simulink model "example_main_NDI_f16"  (R2020a)
settings: Solver=ode4  StartTime=0.0  StopTime=75  FixedStep=0.01  RelTol=1e-3
PreLoadFcn:
  | PreLoadFcn
values from neighbouring files (symbols this model uses):
  g = 32.17    [PreLoadFcn.m]
  N = [ 1      0     0.25 ... (first row only)    [PreLoadFcn.m]
  state0 = [IC.npos IC.epos IC.alt IC.q0 IC.q1 IC.q2 IC.q3  IC.p IC.q IC.r IC.alpha IC.beta IC.mu IC.Vt IC.chi IC.gamma]    [PreLoadFcn.m]
undefined symbols (not defined in the file or in its folder): Aactuator, ac, AeroCoeff, EngineTable, ft, IC, kg, m, Newton, PIController, Raphson, s, sigbuilder_block, slug
libraries: aerolibconvert2 x19, simulink x13, sharedutil x1
(part 1 of 6)
settings Model: Creator=User  LastModifiedBy=user
settings DataIOCC: ReturnWorkspaceOutputs=off
settings DebuggingCC: ArithmeticOperatorsInVariantConditions=warning
settings SFSimCC: CustomCodeUndefinedFunction=UseInterfaceOnly

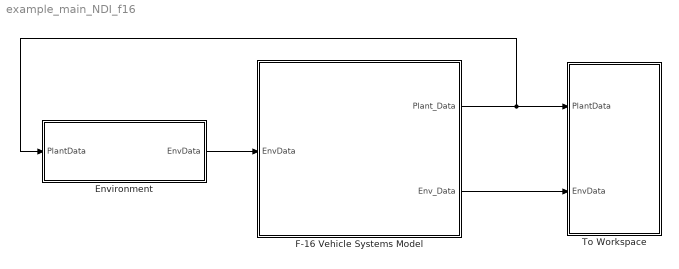
== system example_main_NDI_f16 ==
  Environment : Subsystem
      mask Display:
      | image('aeroenvironment.bmp','center')
      | % 左側 "Icon transparency" 欄位已選擇 "Opaque with ports"，所以埠名稱會自動顯示，不用再宣告
      | % port_label('input',1,'PlantData')
      | % port_label('output',1,'EnvData')
  F-16 Vehicle Systems Model : Subsystem
      mask Display:
      | image([pwd,'\image\wikipedia_F-16.jpg'],'center');
      | % 左側 "Icon transparency" 欄位已選擇 "Opaque with ports"，所以埠名稱會自動顯示，不用再宣告
      | % port_label('input',1,'EnvData')
      | % port_label('output',1,'Plant_Data')
      | % port_label('output',2,'Env_Data')
  To Workspace : Subsystem
  wires:
  F-16 Vehicle Systems Model/1(Plant_Data) -> To Workspace/1(PlantData), Environment/1(PlantData)
  Environment/1(EnvData) -> F-16 Vehicle Systems Model/1(EnvData)
  F-16 Vehicle Systems Model/2(Env_Data) -> To Workspace/2(EnvData)

== system example_main_NDI_f16/Environment ==
  PlantData : Inport
  "ISP " : Subsystem
  end5 : Terminator
  end8 : Terminator
  end9 : Terminator
  gravity (ft/s^2) : Constant  Value=g
  Out Bus Element : Outport  PortName=EnvData  Element=P
  Out Bus Element1 : Outport  PortName=EnvData  Element=AirDensity
  Out Bus Element2 : Outport  PortName=EnvData  Element=qbar
  Out Bus Element3 : Outport  PortName=EnvData  Element=Mach
  Out Bus Element4 : Outport  PortName=EnvData  Element=g
  wires:
  "ISP "/7(mu) -> end9/1
  "ISP "/5(T(K)) -> end5/1
  "ISP "/6(g (m/s^2)) -> end8/1
  PlantData/1 -> "ISP "/1(PlantData)
  "ISP "/1(P(HPa)) -> Out Bus Element/1
  "ISP "/2(rho(kg/m^3)) -> Out Bus Element1/1
  "ISP "/3(qbar (lbf/ft^2)) -> Out Bus Element2/1
  "ISP "/4("Mach ") -> Out Bus Element3/1
  gravity (ft/s^2)/1 -> Out Bus Element4/1  "g"

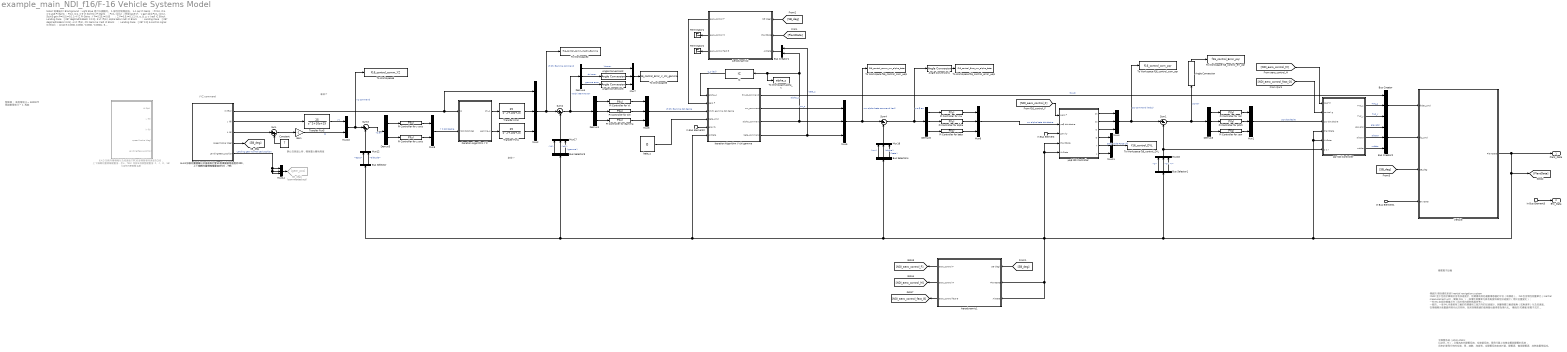
== system example_main_NDI_f16/F-16 Vehicle Systems Model ==
  note: 發動機：
      | 高度限制 0 ~ 50000 ft
      | 馬赫數限制 0 ~ 1 馬赫
  note: 全靜壓系統（pitot-static system），又稱為皮托靜壓系統、空速管系統，是飛行器上收集全壓與靜壓的系統，
      | 用來計算飛行時的空速、馬赫數、海拔等。全靜壓系統由皮托管、靜壓源、備用靜壓源、加熱裝置等組成。
  note: 傳統的 慣性導航系統(inertial navigation system (INS))至少包括計算機及含有加速度計、陀螺儀或其他運動傳感器的平台（或模組）。
      | INS包含慣性測量單元（Inertial measurement unit，簡稱 IMU ），該慣性測量單元具有角度和線性加速度計（用於位置變化）；
      | 一些IMU包括陀螺儀元件（用於保持絕對角度參考）。
      | 一般的，一個IMU內會裝有三軸的陀螺儀和三個方向的加速度計，測量物體三軸姿態角（或角速率）以及加速度。
      |
      | 在飛機顯示裝置變得現代化的同時，為其採集數據的感測器也變得更為現代化。
      | 傳統的 陀螺儀 被電子式的 航向姿態基準系統 （AHRS）與 大氣數據計算機 （ADC）所取代，
      | 在增加可靠性的同時也降低了成本、簡化了維護。
      | 此外， GPS 接收器也被整合進了玻璃駕駛艙之中。
  note: 機載電子設備
  note: 靜止在跑道上時，機身重心離地高度
  note: 拿掉!?
  note: VYZ command
  note: Note:(宥瑋論文)
      | Blockground：Light Blue 是可以調動的。
      | 1.線性控制增益值。
      | 1-1 pqr PI Gains：P=10, I=4.
      | 1-2 μαβ PI Gains：P=2, I=1.
      | 1-3 Vt $\chi$ γ PI Gains：P=1, I=0.2；降落Case:Vt、γ gain設定P=1, I=0.2、 $\chi$ gain P=0.5,I=0.1
      | 1-4 YZ PI Gains : Y P=0.25,I=0.05；Z P=0.5,I=0.1
      | 2.Vt, α, β, μ, γ (rad) IC Block
      | Landing Case：[287 deg2rad(9.8641) 0 0 0].
      | 3.Vt (ft/s), alpha beta (rad) IC Block：
      | Landing Case：[287 deg2rad(9.8641) 0.01].
      | 4.Vt (ft/s), Chi Gamma (rad) IC Block：
      | Landing Case：[287 0 0]
      | 5.control signal IC Block：
      | [2110 5 0.0001 0.0001 -0.0001 -0.0001].
      | 6. 若要在不同高度或是速度下飛行，需重新配平，以配平條件設定初始值。
      | 7. 控制分配權重值需在"pqr NDI Controller/innear NDI"中，N矩陣做調整。
      | 7. 減速板角度調整要在
      | "SB_Aerodynamic_coefficient"、"SB_Aerodynamic_coefficient_2017_iteration"、"SB_Aerodynamic_coefficient_2017_NDI"的m-file檔中做調整。
  note: 拿掉!?
  In Bus Element1 : Inport  PortName=EnvData
  In Bus Element3 : Inport  PortName=EnvData
  In Bus Element : Inport  PortName=EnvData  Element=g
  In Bus Element2 : Inport  PortName=EnvData  Element=g
  6.4.3加裝向量噴嘴以及減速版打開30度模擬著陸速度為200， 上下偏轉向量噴嘴權重值為4，75S (附錄B須調整權重值: 2、4、8、16) : Subsystem  Tag=STV Subsys  Commented=on  LoadFcn=sigbuilder_block('load');  StartFcn=sigbuilder_block('start');  StopFcn=sigbuilder_block('stop');  ClipboardFcn=sigbuilder_block('clipboard');  mask(Sigbuilder block){tuvar=[0:10]}
      mask help: Simulink:masks:SigbuilderBlock_MD
      mask init:
      | if ~strcmp(get_param(bdroot(gcbh),'SimulationStatus'),'stopped') tuvar = sigbuilder_block('maskInit'); end
      settings: CopyFcn=sigbuilder_block('copy');  DeleteFcn=sigbuilder_block('delete');  ModelCloseFcn=sigbuilder_block('modelClose');  PreSaveFcn=sigbuilder_block('preSave');  PauseFcn=sigbuilder_block('pause');  ContinueFcn=sigbuilder_block('continue');  NameChangeFcn=sigbuilder_block('namechange');  OpenFcn=sigbuilder_block('open',[6 30 1428 680.25 ]);  CloseFcn=sigbuilder_block('close');
      mask Display: plot(0, 0, 100, 100,[2, 2, 32, 32, 2], [68, 8, 8, 68, 68],[32, 2], [38, 38], [32, 19, 2],[53, 60, 44], [32, 17, 17, 2],[16, 16, 31, 31]);txt = getActiveGroup(gcbh);text(2, 100, txt,'verticalAlignment', 'top');
  6.4.3加裝向量噴嘴以及減速版打開40度模擬著陸速度為200， 上下偏轉向量噴嘴權重值為5.5，75S : Subsystem  Tag=STV Subsys  LoadFcn=sigbuilder_block('load');  StartFcn=sigbuilder_block('start');  StopFcn=sigbuilder_block('stop');  ClipboardFcn=sigbuilder_block('clipboard');  mask(Sigbuilder block){tuvar=[0:10]}
      mask help: Simulink:masks:SigbuilderBlock_MD
      mask init:
      | if ~strcmp(get_param(bdroot(gcbh),'SimulationStatus'),'stopped') tuvar = sigbuilder_block('maskInit'); end
      settings: CopyFcn=sigbuilder_block('copy');  DeleteFcn=sigbuilder_block('delete');  ModelCloseFcn=sigbuilder_block('modelClose');  PreSaveFcn=sigbuilder_block('preSave');  PauseFcn=sigbuilder_block('pause');  ContinueFcn=sigbuilder_block('continue');  NameChangeFcn=sigbuilder_block('namechange');  OpenFcn=sigbuilder_block('open',[6 30 1428 680.25 ]);  CloseFcn=sigbuilder_block('close');
      mask Display: plot(0, 0, 100, 100,[2, 2, 32, 32, 2], [68, 8, 8, 68, 68],[32, 2], [38, 38], [32, 19, 2],[53, 60, 44], [32, 17, 17, 2],[16, 16, 31, 31]);txt = getActiveGroup(gcbh);text(2, 100, txt,'verticalAlignment', 'top');
  Aerodynamic1 : Subsystem
  Aerodynamic2 : Subsystem
  Angle Conversion{,1..3} (4 alike) : aerolibconvert2/Angle Conversion  IU=rad  OU=deg
  Bus Creator : BusCreator  Inputs=3
  Bus Creator1 : BusCreator  Inputs=2
  Bus Creator2 : BusCreator  Inputs=3
  Bus Selector : BusSelector  OutputSignals=epos,altitude
  Bus Selector1 : BusSelector  OutputSignals=p,q,r
  Bus Selector3 : BusSelector  OutputSignals=Vt,chi,gamma
  Bus Selector4 : BusSelector  OutputSignals=mu,alpha,beta
  Constant : Constant  Value=7
  Demux{1,3..4,6} (4 alike) : Demux  Outputs=3
  Demux5 : Demux  Outputs=2
  Gain : Gain  Gain=-1
  IC : InitialCondition  Value=IC.alpha
  Iteration Algorithm V chi gamma : Subsystem
  Iteration Algorithm Y Z : Subsystem
  Mux{1..7,11,14,16..18} (12 alike) : Mux  Inputs=3
  Mux10 : Mux  Inputs=2
  Mux12 : Mux  Inputs=2
  Mux9 : Mux  Inputs=2
  PI Controller for Chi : simulink/Continuous/PID Controller  Controller=PI  Form=Parallel  TimeDomain=Continuous-time  UseExternalTs=off  SampleTime=-1  IntegratorMethod=Forward Euler  FilterMethod=Forward Euler  ControllerParametersSource=internal  P=PIController.chi.P  I=PIController.chi.I  D=0  UseFilter=on  N=100  TunerSelectOption=Transfer Function Based (PID Tuner App)  InitialConditionSource=internal  InitialConditionForIntegrator=0  InitialConditionForFilter=0  DifferentiatorICPrevScaledInput=0  ExternalReset=none  TrackingMode=off  Kt=1  LimitOutput=off  UpperSaturationLimit=inf  LowerSaturationLimit=-inf  LinearizeAsGain=on  AntiWindupMode=none  Kb=1  POutMin=[]  POutMax=[]  IOutMin=[]  IOutMax=[]  DOutMin=[]  DOutMax=[]  NOutMin=[]  NOutMax=[]  SumOutMin=[]  SumOutMax=[]  SaturationOutMin=[]  SaturationOutMax=[]  PParamMin=[]  PParamMax=[]  IParamMin=[]  IParamMax=[]  DParamMin=[]  DParamMax=[]  NParamMin=[]  NParamMax=[]  KbParamMin=[]  KbParamMax=[]  KtParamMin=[]  KtParamMax=[]  KbOutMin=[]  KbOutMax=[]  KtOutMin=[]  KtOutMax=[]  IntegratorOutMin=[]  IntegratorOutMax=[]  FilterOutMin=[]  FilterOutMax=[]  SumI1OutMin=[]  SumI1OutMax=[]  SumI2OutMin=[]  SumI2OutMax=[]  SumI3OutMin=[]  SumI3OutMax=[]  SumI4OutMin=[]  SumI4OutMax=[]  SumDOutMin=[]  SumDOutMax=[]  DifferentiatorOutMin=[]  DifferentiatorOutMax=[]  FilterDiffOutCoefMin=[]  FilterDiffOutCoefMax=[]  ReciprocalOutMin=[]  ReciprocalOutMax=[]  SumDenOutMin=[]  SumDenOutMax=[]  SumNumOutMin=[]  SumNumOutMax=[]  DivideOutMin=[]  DivideOutMax=[]  UdiffTsProdOutMin=[]  UdiffTsProdOutMax=[]  NTsProdOutMin=[]  NTsProdOutMax=[]  UintegralTsProdOutMin=[]  UintegralTsProdOutMax=[]  UngainTsProdOutMin=[]  UngainTsProdOutMax=[]  IntegratorContinuousStateAttributes=''  IntegratorStateMustResolveToSignalObject=off  IntegratorRTWStateStorageClass=Auto  FilterContinuousStateAttributes=''  FilterStateMustResolveToSignalObject=off  FilterRTWStateStorageClass=Auto  ParallelPVariant=InternalParameters  IdealPVariant=Disabled  IVariant=InternalParameters  DVariant=Disabled  IntegratorVariant=Continuous  SatVariant=Disabled  AWVariant=Passthrough  PCopyVariant=Disabled  TRVariant=Disabled  FdbkBlocksVariant=Forward  IdealPFdbkVariant=Disabled  SatFdbkVariant=Disabled  DerivativeFilterVariant=Disabled  NVariant=Disabled  NCopyVariant=Disabled_SignalSpec  FilterICVariant=Disabled  IntegratorICVariant=InternalICs  ExternalResetVariant=Disabled  TRSumVariant=Passthrough  SumFdbkVariant=Disabled  SumVariant=Sum_PI  TsampFilterVariant=InternalTs  TsampNgainVariant=Passthrough  TsampIntegralVariant=Passthrough
  PI Controller for Gamma : simulink/Continuous/PID Controller  Controller=PI  Form=Parallel  TimeDomain=Continuous-time  UseExternalTs=off  SampleTime=-1  IntegratorMethod=Forward Euler  FilterMethod=Forward Euler  ControllerParametersSource=internal  P=PIController.gamma.P  I=PIController.gamma.I  D=0  UseFilter=on  N=100  TunerSelectOption=Transfer Function Based (PID Tuner App)  InitialConditionSource=internal  InitialConditionForIntegrator=0  InitialConditionForFilter=0  DifferentiatorICPrevScaledInput=0  ExternalReset=none  TrackingMode=off  Kt=1  LimitOutput=off  UpperSaturationLimit=inf  LowerSaturationLimit=-inf  LinearizeAsGain=on  AntiWindupMode=none  Kb=1  POutMin=[]  POutMax=[]  IOutMin=[]  IOutMax=[]  DOutMin=[]  DOutMax=[]  NOutMin=[]  NOutMax=[]  SumOutMin=[]  SumOutMax=[]  SaturationOutMin=[]  SaturationOutMax=[]  PParamMin=[]  PParamMax=[]  IParamMin=[]  IParamMax=[]  DParamMin=[]  DParamMax=[]  NParamMin=[]  NParamMax=[]  KbParamMin=[]  KbParamMax=[]  KtParamMin=[]  KtParamMax=[]  KbOutMin=[]  KbOutMax=[]  KtOutMin=[]  KtOutMax=[]  IntegratorOutMin=[]  IntegratorOutMax=[]  FilterOutMin=[]  FilterOutMax=[]  SumI1OutMin=[]  SumI1OutMax=[]  SumI2OutMin=[]  SumI2OutMax=[]  SumI3OutMin=[]  SumI3OutMax=[]  SumI4OutMin=[]  SumI4OutMax=[]  SumDOutMin=[]  SumDOutMax=[]  DifferentiatorOutMin=[]  DifferentiatorOutMax=[]  FilterDiffOutCoefMin=[]  FilterDiffOutCoefMax=[]  ReciprocalOutMin=[]  ReciprocalOutMax=[]  SumDenOutMin=[]  SumDenOutMax=[]  SumNumOutMin=[]  SumNumOutMax=[]  DivideOutMin=[]  DivideOutMax=[]  UdiffTsProdOutMin=[]  UdiffTsProdOutMax=[]  NTsProdOutMin=[]  NTsProdOutMax=[]  UintegralTsProdOutMin=[]  UintegralTsProdOutMax=[]  UngainTsProdOutMin=[]  UngainTsProdOutMax=[]  IntegratorContinuousStateAttributes=''  IntegratorStateMustResolveToSignalObject=off  IntegratorRTWStateStorageClass=Auto  FilterContinuousStateAttributes=''  FilterStateMustResolveToSignalObject=off  FilterRTWStateStorageClass=Auto  ParallelPVariant=InternalParameters  IdealPVariant=Disabled  IVariant=InternalParameters  DVariant=Disabled  IntegratorVariant=Continuous  SatVariant=Disabled  AWVariant=Passthrough  PCopyVariant=Disabled  TRVariant=Disabled  FdbkBlocksVariant=Forward  IdealPFdbkVariant=Disabled  SatFdbkVariant=Disabled  DerivativeFilterVariant=Disabled  NVariant=Disabled  NCopyVariant=Disabled_SignalSpec  FilterICVariant=Disabled  IntegratorICVariant=InternalICs  ExternalResetVariant=Disabled  TRSumVariant=Passthrough  SumFdbkVariant=Disabled  SumVariant=Sum_PI  TsampFilterVariant=InternalTs  TsampNgainVariant=Passthrough  TsampIntegralVariant=Passthrough
  PI Controller for Vt : simulink/Continuous/PID Controller  Controller=PI  Form=Parallel  TimeDomain=Continuous-time  UseExternalTs=off  SampleTime=-1  IntegratorMethod=Forward Euler  FilterMethod=Forward Euler  ControllerParametersSource=internal  P=PIController.Vt.P  I=PIController.Vt.I  D=0  UseFilter=on  N=100  TunerSelectOption=Transfer Function Based (PID Tuner App)  InitialConditionSource=internal  InitialConditionForIntegrator=0  InitialConditionForFilter=0  DifferentiatorICPrevScaledInput=0  ExternalReset=none  TrackingMode=off  Kt=1  LimitOutput=off  UpperSaturationLimit=inf  LowerSaturationLimit=-inf  LinearizeAsGain=on  AntiWindupMode=none  Kb=1  POutMin=[]  POutMax=[]  IOutMin=[]  IOutMax=[]  DOutMin=[]  DOutMax=[]  NOutMin=[]  NOutMax=[]  SumOutMin=[]  SumOutMax=[]  SaturationOutMin=[]  SaturationOutMax=[]  PParamMin=[]  PParamMax=[]  IParamMin=[]  IParamMax=[]  DParamMin=[]  DParamMax=[]  NParamMin=[]  NParamMax=[]  KbParamMin=[]  KbParamMax=[]  KtParamMin=[]  KtParamMax=[]  KbOutMin=[]  KbOutMax=[]  KtOutMin=[]  KtOutMax=[]  IntegratorOutMin=[]  IntegratorOutMax=[]  FilterOutMin=[]  FilterOutMax=[]  SumI1OutMin=[]  SumI1OutMax=[]  SumI2OutMin=[]  SumI2OutMax=[]  SumI3OutMin=[]  SumI3OutMax=[]  SumI4OutMin=[]  SumI4OutMax=[]  SumDOutMin=[]  SumDOutMax=[]  DifferentiatorOutMin=[]  DifferentiatorOutMax=[]  FilterDiffOutCoefMin=[]  FilterDiffOutCoefMax=[]  ReciprocalOutMin=[]  ReciprocalOutMax=[]  SumDenOutMin=[]  SumDenOutMax=[]  SumNumOutMin=[]  SumNumOutMax=[]  DivideOutMin=[]  DivideOutMax=[]  UdiffTsProdOutMin=[]  UdiffTsProdOutMax=[]  NTsProdOutMin=[]  NTsProdOutMax=[]  UintegralTsProdOutMin=[]  UintegralTsProdOutMax=[]  UngainTsProdOutMin=[]  UngainTsProdOutMax=[]  IntegratorContinuousStateAttributes=''  IntegratorStateMustResolveToSignalObject=off  IntegratorRTWStateStorageClass=Auto  FilterContinuousStateAttributes=''  FilterStateMustResolveToSignalObject=off  FilterRTWStateStorageClass=Auto  ParallelPVariant=InternalParameters  IdealPVariant=Disabled  IVariant=InternalParameters  DVariant=Disabled  IntegratorVariant=Continuous  SatVariant=Disabled  AWVariant=Passthrough  PCopyVariant=Disabled  TRVariant=Disabled  FdbkBlocksVariant=Forward  IdealPFdbkVariant=Disabled  SatFdbkVariant=Disabled  DerivativeFilterVariant=Disabled  NVariant=Disabled  NCopyVariant=Disabled_SignalSpec  FilterICVariant=Disabled  IntegratorICVariant=InternalICs  ExternalResetVariant=Disabled  TRSumVariant=Passthrough  SumFdbkVariant=Disabled  SumVariant=Sum_PI  TsampFilterVariant=InternalTs  TsampNgainVariant=Passthrough  TsampIntegralVariant=Passthrough
  PI Controller for alpha : simulink/Continuous/PID Controller  Controller=PI  Form=Parallel  TimeDomain=Continuous-time  UseExternalTs=off  SampleTime=-1  IntegratorMethod=Forward Euler  FilterMethod=Forward Euler  ControllerParametersSource=internal  P=PIController.alpha.P  I=PIController.alpha.I  D=0  UseFilter=on  N=100  TunerSelectOption=Transfer Function Based (PID Tuner App)  InitialConditionSource=internal  InitialConditionForIntegrator=0  InitialConditionForFilter=0  DifferentiatorICPrevScaledInput=0  ExternalReset=none  TrackingMode=off  Kt=1  LimitOutput=off  UpperSaturationLimit=inf  LowerSaturationLimit=-inf  LinearizeAsGain=on  AntiWindupMode=none  Kb=1  POutMin=[]  POutMax=[]  IOutMin=[]  IOutMax=[]  DOutMin=[]  DOutMax=[]  NOutMin=[]  NOutMax=[]  SumOutMin=[]  SumOutMax=[]  SaturationOutMin=[]  SaturationOutMax=[]  PParamMin=[]  PParamMax=[]  IParamMin=[]  IParamMax=[]  DParamMin=[]  DParamMax=[]  NParamMin=[]  NParamMax=[]  KbParamMin=[]  KbParamMax=[]  KtParamMin=[]  KtParamMax=[]  KbOutMin=[]  KbOutMax=[]  KtOutMin=[]  KtOutMax=[]  IntegratorOutMin=[]  IntegratorOutMax=[]  FilterOutMin=[]  FilterOutMax=[]  SumI1OutMin=[]  SumI1OutMax=[]  SumI2OutMin=[]  SumI2OutMax=[]  SumI3OutMin=[]  SumI3OutMax=[]  SumI4OutMin=[]  SumI4OutMax=[]  SumDOutMin=[]  SumDOutMax=[]  DifferentiatorOutMin=[]  DifferentiatorOutMax=[]  FilterDiffOutCoefMin=[]  FilterDiffOutCoefMax=[]  ReciprocalOutMin=[]  ReciprocalOutMax=[]  SumDenOutMin=[]  SumDenOutMax=[]  SumNumOutMin=[]  SumNumOutMax=[]  DivideOutMin=[]  DivideOutMax=[]  UdiffTsProdOutMin=[]  UdiffTsProdOutMax=[]  NTsProdOutMin=[]  NTsProdOutMax=[]  UintegralTsProdOutMin=[]  UintegralTsProdOutMax=[]  UngainTsProdOutMin=[]  UngainTsProdOutMax=[]  IntegratorContinuousStateAttributes=''  IntegratorStateMustResolveToSignalObject=off  IntegratorRTWStateStorageClass=Auto  FilterContinuousStateAttributes=''  FilterStateMustResolveToSignalObject=off  FilterRTWStateStorageClass=Auto  ParallelPVariant=InternalParameters  IdealPVariant=Disabled  IVariant=InternalParameters  DVariant=Disabled  IntegratorVariant=Continuous  SatVariant=Disabled  AWVariant=Passthrough  PCopyVariant=Disabled  TRVariant=Disabled  FdbkBlocksVariant=Forward  IdealPFdbkVariant=Disabled  SatFdbkVariant=Disabled  DerivativeFilterVariant=Disabled  NVariant=Disabled  NCopyVariant=Disabled_SignalSpec  FilterICVariant=Disabled  IntegratorICVariant=InternalICs  ExternalResetVariant=Disabled  TRSumVariant=Passthrough  SumFdbkVariant=Disabled  SumVariant=Sum_PI  TsampFilterVariant=InternalTs  TsampNgainVariant=Passthrough  TsampIntegralVariant=Passthrough
  PI Controller for beta : simulink/Continuous/PID Controller  Controller=PI  Form=Parallel  TimeDomain=Continuous-time  UseExternalTs=off  SampleTime=-1  IntegratorMethod=Forward Euler  FilterMethod=Forward Euler  ControllerParametersSource=internal  P=PIController.beta.P  I=PIController.beta.I  D=0  UseFilter=on  N=100  TunerSelectOption=Transfer Function Based (PID Tuner App)  InitialConditionSource=internal  InitialConditionForIntegrator=0  InitialConditionForFilter=0  DifferentiatorICPrevScaledInput=0  ExternalReset=none  TrackingMode=off  Kt=1  LimitOutput=off  UpperSaturationLimit=inf  LowerSaturationLimit=-inf  LinearizeAsGain=on  AntiWindupMode=none  Kb=1  POutMin=[]  POutMax=[]  IOutMin=[]  IOutMax=[]  DOutMin=[]  DOutMax=[]  NOutMin=[]  NOutMax=[]  SumOutMin=[]  SumOutMax=[]  SaturationOutMin=[]  SaturationOutMax=[]  PParamMin=[]  PParamMax=[]  IParamMin=[]  IParamMax=[]  DParamMin=[]  DParamMax=[]  NParamMin=[]  NParamMax=[]  KbParamMin=[]  KbParamMax=[]  KtParamMin=[]  KtParamMax=[]  KbOutMin=[]  KbOutMax=[]  KtOutMin=[]  KtOutMax=[]  IntegratorOutMin=[]  IntegratorOutMax=[]  FilterOutMin=[]  FilterOutMax=[]  SumI1OutMin=[]  SumI1OutMax=[]  SumI2OutMin=[]  SumI2OutMax=[]  SumI3OutMin=[]  SumI3OutMax=[]  SumI4OutMin=[]  SumI4OutMax=[]  SumDOutMin=[]  SumDOutMax=[]  DifferentiatorOutMin=[]  DifferentiatorOutMax=[]  FilterDiffOutCoefMin=[]  FilterDiffOutCoefMax=[]  ReciprocalOutMin=[]  ReciprocalOutMax=[]  SumDenOutMin=[]  SumDenOutMax=[]  SumNumOutMin=[]  SumNumOutMax=[]  DivideOutMin=[]  DivideOutMax=[]  UdiffTsProdOutMin=[]  UdiffTsProdOutMax=[]  NTsProdOutMin=[]  NTsProdOutMax=[]  UintegralTsProdOutMin=[]  UintegralTsProdOutMax=[]  UngainTsProdOutMin=[]  UngainTsProdOutMax=[]  IntegratorContinuousStateAttributes=''  IntegratorStateMustResolveToSignalObject=off  IntegratorRTWStateStorageClass=Auto  FilterContinuousStateAttributes=''  FilterStateMustResolveToSignalObject=off  FilterRTWStateStorageClass=Auto  ParallelPVariant=InternalParameters  IdealPVariant=Disabled  IVariant=InternalParameters  DVariant=Disabled  IntegratorVariant=Continuous  SatVariant=Disabled  AWVariant=Passthrough  PCopyVariant=Disabled  TRVariant=Disabled  FdbkBlocksVariant=Forward  IdealPFdbkVariant=Disabled  SatFdbkVariant=Disabled  DerivativeFilterVariant=Disabled  NVariant=Disabled  NCopyVariant=Disabled_SignalSpec  FilterICVariant=Disabled  IntegratorICVariant=InternalICs  ExternalResetVariant=Disabled  TRSumVariant=Passthrough  SumFdbkVariant=Disabled  SumVariant=Sum_PI  TsampFilterVariant=InternalTs  TsampNgainVariant=Passthrough  TsampIntegralVariant=Passthrough
  PI Controller for mu : simulink/Continuous/PID Controller  Controller=PI  Form=Parallel  TimeDomain=Continuous-time  UseExternalTs=off  SampleTime=-1  IntegratorMethod=Forward Euler  FilterMethod=Forward Euler  ControllerParametersSource=internal  P=PIController.mu.P  I=PIController.mu.I  D=0  UseFilter=on  N=100  TunerSelectOption=Transfer Function Based (PID Tuner App)  InitialConditionSource=internal  InitialConditionForIntegrator=0  InitialConditionForFilter=0  DifferentiatorICPrevScaledInput=0  ExternalReset=none  TrackingMode=off  Kt=1  LimitOutput=off  UpperSaturationLimit=inf  LowerSaturationLimit=-inf  LinearizeAsGain=on  AntiWindupMode=none  Kb=1  POutMin=[]  POutMax=[]  IOutMin=[]  IOutMax=[]  DOutMin=[]  DOutMax=[]  NOutMin=[]  NOutMax=[]  SumOutMin=[]  SumOutMax=[]  SaturationOutMin=[]  SaturationOutMax=[]  PParamMin=[]  PParamMax=[]  IParamMin=[]  IParamMax=[]  DParamMin=[]  DParamMax=[]  NParamMin=[]  NParamMax=[]  KbParamMin=[]  KbParamMax=[]  KtParamMin=[]  KtParamMax=[]  KbOutMin=[]  KbOutMax=[]  KtOutMin=[]  KtOutMax=[]  IntegratorOutMin=[]  IntegratorOutMax=[]  FilterOutMin=[]  FilterOutMax=[]  SumI1OutMin=[]  SumI1OutMax=[]  SumI2OutMin=[]  SumI2OutMax=[]  SumI3OutMin=[]  SumI3OutMax=[]  SumI4OutMin=[]  SumI4OutMax=[]  SumDOutMin=[]  SumDOutMax=[]  DifferentiatorOutMin=[]  DifferentiatorOutMax=[]  FilterDiffOutCoefMin=[]  FilterDiffOutCoefMax=[]  ReciprocalOutMin=[]  ReciprocalOutMax=[]  SumDenOutMin=[]  SumDenOutMax=[]  SumNumOutMin=[]  SumNumOutMax=[]  DivideOutMin=[]  DivideOutMax=[]  UdiffTsProdOutMin=[]  UdiffTsProdOutMax=[]  NTsProdOutMin=[]  NTsProdOutMax=[]  UintegralTsProdOutMin=[]  UintegralTsProdOutMax=[]  UngainTsProdOutMin=[]  UngainTsProdOutMax=[]  IntegratorContinuousStateAttributes=''  IntegratorStateMustResolveToSignalObject=off  IntegratorRTWStateStorageClass=Auto  FilterContinuousStateAttributes=''  FilterStateMustResolveToSignalObject=off  FilterRTWStateStorageClass=Auto  ParallelPVariant=InternalParameters  IdealPVariant=Disabled  IVariant=InternalParameters  DVariant=Disabled  IntegratorVariant=Continuous  SatVariant=Disabled  AWVariant=Passthrough  PCopyVariant=Disabled  TRVariant=Disabled  FdbkBlocksVariant=Forward  IdealPFdbkVariant=Disabled  SatFdbkVariant=Disabled  DerivativeFilterVariant=Disabled  NVariant=Disabled  NCopyVariant=Disabled_SignalSpec  FilterICVariant=Disabled  IntegratorICVariant=InternalICs  ExternalResetVariant=Disabled  TRSumVariant=Passthrough  SumFdbkVariant=Disabled  SumVariant=Sum_PI  TsampFilterVariant=InternalTs  TsampNgainVariant=Passthrough  TsampIntegralVariant=Passthrough
  PI Controller for pitch : simulink/Continuous/PID Controller  Controller=PI  Form=Parallel  TimeDomain=Continuous-time  UseExternalTs=off  SampleTime=-1  IntegratorMethod=Forward Euler  FilterMethod=Forward Euler  ControllerParametersSource=internal  P=PIController.q.P  I=PIController.q.I  D=0  UseFilter=on  N=100  TunerSelectOption=Transfer Function Based (PID Tuner App)  InitialConditionSource=internal  InitialConditionForIntegrator=0  InitialConditionForFilter=0  DifferentiatorICPrevScaledInput=0  ExternalReset=none  TrackingMode=off  Kt=1  LimitOutput=off  UpperSaturationLimit=inf  LowerSaturationLimit=-inf  LinearizeAsGain=on  AntiWindupMode=none  Kb=1  POutMin=[]  POutMax=[]  IOutMin=[]  IOutMax=[]  DOutMin=[]  DOutMax=[]  NOutMin=[]  NOutMax=[]  SumOutMin=[]  SumOutMax=[]  SaturationOutMin=[]  SaturationOutMax=[]  PParamMin=[]  PParamMax=[]  IParamMin=[]  IParamMax=[]  DParamMin=[]  DParamMax=[]  NParamMin=[]  NParamMax=[]  KbParamMin=[]  KbParamMax=[]  KtParamMin=[]  KtParamMax=[]  KbOutMin=[]  KbOutMax=[]  KtOutMin=[]  KtOutMax=[]  IntegratorOutMin=[]  IntegratorOutMax=[]  FilterOutMin=[]  FilterOutMax=[]  SumI1OutMin=[]  SumI1OutMax=[]  SumI2OutMin=[]  SumI2OutMax=[]  SumI3OutMin=[]  SumI3OutMax=[]  SumI4OutMin=[]  SumI4OutMax=[]  SumDOutMin=[]  SumDOutMax=[]  DifferentiatorOutMin=[]  DifferentiatorOutMax=[]  FilterDiffOutCoefMin=[]  FilterDiffOutCoefMax=[]  ReciprocalOutMin=[]  ReciprocalOutMax=[]  SumDenOutMin=[]  SumDenOutMax=[]  SumNumOutMin=[]  SumNumOutMax=[]  DivideOutMin=[]  DivideOutMax=[]  UdiffTsProdOutMin=[]  UdiffTsProdOutMax=[]  NTsProdOutMin=[]  NTsProdOutMax=[]  UintegralTsProdOutMin=[]  UintegralTsProdOutMax=[]  UngainTsProdOutMin=[]  UngainTsProdOutMax=[]  IntegratorContinuousStateAttributes=''  IntegratorStateMustResolveToSignalObject=off  IntegratorRTWStateStorageClass=Auto  FilterContinuousStateAttributes=''  FilterStateMustResolveToSignalObject=off  FilterRTWStateStorageClass=Auto  ParallelPVariant=InternalParameters  IdealPVariant=Disabled  IVariant=InternalParameters  DVariant=Disabled  IntegratorVariant=Continuous  SatVariant=Disabled  AWVariant=Passthrough  PCopyVariant=Disabled  TRVariant=Disabled  FdbkBlocksVariant=Forward  IdealPFdbkVariant=Disabled  SatFdbkVariant=Disabled  DerivativeFilterVariant=Disabled  NVariant=Disabled  NCopyVariant=Disabled_SignalSpec  FilterICVariant=Disabled  IntegratorICVariant=InternalICs  ExternalResetVariant=Disabled  TRSumVariant=Passthrough  SumFdbkVariant=Disabled  SumVariant=Sum_PI  TsampFilterVariant=InternalTs  TsampNgainVariant=Passthrough  TsampIntegralVariant=Passthrough
  PI Controller for roll : simulink/Continuous/PID Controller  Controller=PI  Form=Parallel  TimeDomain=Continuous-time  UseExternalTs=off  SampleTime=-1  IntegratorMethod=Forward Euler  FilterMethod=Forward Euler  ControllerParametersSource=internal  P=PIController.p.P  I=PIController.p.I  D=0  UseFilter=on  N=100  TunerSelectOption=Transfer Function Based (PID Tuner App)  InitialConditionSource=internal  InitialConditionForIntegrator=0  InitialConditionForFilter=0  DifferentiatorICPrevScaledInput=0  ExternalReset=none  TrackingMode=off  Kt=1  LimitOutput=off  UpperSaturationLimit=inf  LowerSaturationLimit=-inf  LinearizeAsGain=on  AntiWindupMode=none  Kb=1  POutMin=[]  POutMax=[]  IOutMin=[]  IOutMax=[]  DOutMin=[]  DOutMax=[]  NOutMin=[]  NOutMax=[]  SumOutMin=[]  SumOutMax=[]  SaturationOutMin=[]  SaturationOutMax=[]  PParamMin=[]  PParamMax=[]  IParamMin=[]  IParamMax=[]  DParamMin=[]  DParamMax=[]  NParamMin=[]  NParamMax=[]  KbParamMin=[]  KbParamMax=[]  KtParamMin=[]  KtParamMax=[]  KbOutMin=[]  KbOutMax=[]  KtOutMin=[]  KtOutMax=[]  IntegratorOutMin=[]  IntegratorOutMax=[]  FilterOutMin=[]  FilterOutMax=[]  SumI1OutMin=[]  SumI1OutMax=[]  SumI2OutMin=[]  SumI2OutMax=[]  SumI3OutMin=[]  SumI3OutMax=[]  SumI4OutMin=[]  SumI4OutMax=[]  SumDOutMin=[]  SumDOutMax=[]  DifferentiatorOutMin=[]  DifferentiatorOutMax=[]  FilterDiffOutCoefMin=[]  FilterDiffOutCoefMax=[]  ReciprocalOutMin=[]  ReciprocalOutMax=[]  SumDenOutMin=[]  SumDenOutMax=[]  SumNumOutMin=[]  SumNumOutMax=[]  DivideOutMin=[]  DivideOutMax=[]  UdiffTsProdOutMin=[]  UdiffTsProdOutMax=[]  NTsProdOutMin=[]  NTsProdOutMax=[]  UintegralTsProdOutMin=[]  UintegralTsProdOutMax=[]  UngainTsProdOutMin=[]  UngainTsProdOutMax=[]  IntegratorContinuousStateAttributes=''  IntegratorStateMustResolveToSignalObject=off  IntegratorRTWStateStorageClass=Auto  FilterContinuousStateAttributes=''  FilterStateMustResolveToSignalObject=off  FilterRTWStateStorageClass=Auto  ParallelPVariant=InternalParameters  IdealPVariant=Disabled  IVariant=InternalParameters  DVariant=Disabled  IntegratorVariant=Continuous  SatVariant=Disabled  AWVariant=Passthrough  PCopyVariant=Disabled  TRVariant=Disabled  FdbkBlocksVariant=Forward  IdealPFdbkVariant=Disabled  SatFdbkVariant=Disabled  DerivativeFilterVariant=Disabled  NVariant=Disabled  NCopyVariant=Disabled_SignalSpec  FilterICVariant=Disabled  IntegratorICVariant=InternalICs  ExternalResetVariant=Disabled  TRSumVariant=Passthrough  SumFdbkVariant=Disabled  SumVariant=Sum_PI  TsampFilterVariant=InternalTs  TsampNgainVariant=Passthrough  TsampIntegralVariant=Passthrough
  PI Controller for y axis : simulink/Continuous/PID Controller  Controller=PI  Form=Parallel  TimeDomain=Continuous-time  UseExternalTs=off  SampleTime=-1  IntegratorMethod=Forward Euler  FilterMethod=Forward Euler  ControllerParametersSource=internal  P=PIController.y.P  I=PIController.y.I  D=0  UseFilter=on  N=100  TunerSelectOption=Transfer Function Based (PID Tuner App)  InitialConditionSource=internal  InitialConditionForIntegrator=0  InitialConditionForFilter=0  DifferentiatorICPrevScaledInput=0  ExternalReset=none  TrackingMode=off  Kt=1  LimitOutput=off  UpperSaturationLimit=inf  LowerSaturationLimit=-inf  LinearizeAsGain=on  AntiWindupMode=none  Kb=1  POutMin=[]  POutMax=[]  IOutMin=[]  IOutMax=[]  DOutMin=[]  DOutMax=[]  NOutMin=[]  NOutMax=[]  SumOutMin=[]  SumOutMax=[]  SaturationOutMin=[]  SaturationOutMax=[]  PParamMin=[]  PParamMax=[]  IParamMin=[]  IParamMax=[]  DParamMin=[]  DParamMax=[]  NParamMin=[]  NParamMax=[]  KbParamMin=[]  KbParamMax=[]  KtParamMin=[]  KtParamMax=[]  KbOutMin=[]  KbOutMax=[]  KtOutMin=[]  KtOutMax=[]  IntegratorOutMin=[]  IntegratorOutMax=[]  FilterOutMin=[]  FilterOutMax=[]  SumI1OutMin=[]  SumI1OutMax=[]  SumI2OutMin=[]  SumI2OutMax=[]  SumI3OutMin=[]  SumI3OutMax=[]  SumI4OutMin=[]  SumI4OutMax=[]  SumDOutMin=[]  SumDOutMax=[]  DifferentiatorOutMin=[]  DifferentiatorOutMax=[]  FilterDiffOutCoefMin=[]  FilterDiffOutCoefMax=[]  ReciprocalOutMin=[]  ReciprocalOutMax=[]  SumDenOutMin=[]  SumDenOutMax=[]  SumNumOutMin=[]  SumNumOutMax=[]  DivideOutMin=[]  DivideOutMax=[]  UdiffTsProdOutMin=[]  UdiffTsProdOutMax=[]  NTsProdOutMin=[]  NTsProdOutMax=[]  UintegralTsProdOutMin=[]  UintegralTsProdOutMax=[]  UngainTsProdOutMin=[]  UngainTsProdOutMax=[]  IntegratorContinuousStateAttributes=''  IntegratorStateMustResolveToSignalObject=off  IntegratorRTWStateStorageClass=Auto  FilterContinuousStateAttributes=''  FilterStateMustResolveToSignalObject=off  FilterRTWStateStorageClass=Auto  ParallelPVariant=InternalParameters  IdealPVariant=Disabled  IVariant=InternalParameters  DVariant=Disabled  IntegratorVariant=Continuous  SatVariant=Disabled  AWVariant=Passthrough  PCopyVariant=Disabled  TRVariant=Disabled  FdbkBlocksVariant=Forward  IdealPFdbkVariant=Disabled  SatFdbkVariant=Disabled  DerivativeFilterVariant=Disabled  NVariant=Disabled  NCopyVariant=Disabled_SignalSpec  FilterICVariant=Disabled  IntegratorICVariant=InternalICs  ExternalResetVariant=Disabled  TRSumVariant=Passthrough  SumFdbkVariant=Disabled  SumVariant=Sum_PI  TsampFilterVariant=InternalTs  TsampNgainVariant=Passthrough  TsampIntegralVariant=Passthrough
  PI Controller for yaw : simulink/Continuous/PID Controller  Controller=PI  Form=Parallel  TimeDomain=Continuous-time  UseExternalTs=off  SampleTime=-1  IntegratorMethod=Forward Euler  FilterMethod=Forward Euler  ControllerParametersSource=internal  P=PIController.r.P  I=PIController.r.I  D=0  UseFilter=on  N=100  TunerSelectOption=Transfer Function Based (PID Tuner App)  InitialConditionSource=internal  InitialConditionForIntegrator=0  InitialConditionForFilter=0  DifferentiatorICPrevScaledInput=0  ExternalReset=none  TrackingMode=off  Kt=1  LimitOutput=off  UpperSaturationLimit=inf  LowerSaturationLimit=-inf  LinearizeAsGain=on  AntiWindupMode=none  Kb=1  POutMin=[]  POutMax=[]  IOutMin=[]  IOutMax=[]  DOutMin=[]  DOutMax=[]  NOutMin=[]  NOutMax=[]  SumOutMin=[]  SumOutMax=[]  SaturationOutMin=[]  SaturationOutMax=[]  PParamMin=[]  PParamMax=[]  IParamMin=[]  IParamMax=[]  DParamMin=[]  DParamMax=[]  NParamMin=[]  NParamMax=[]  KbParamMin=[]  KbParamMax=[]  KtParamMin=[]  KtParamMax=[]  KbOutMin=[]  KbOutMax=[]  KtOutMin=[]  KtOutMax=[]  IntegratorOutMin=[]  IntegratorOutMax=[]  FilterOutMin=[]  FilterOutMax=[]  SumI1OutMin=[]  SumI1OutMax=[]  SumI2OutMin=[]  SumI2OutMax=[]  SumI3OutMin=[]  SumI3OutMax=[]  SumI4OutMin=[]  SumI4OutMax=[]  SumDOutMin=[]  SumDOutMax=[]  DifferentiatorOutMin=[]  DifferentiatorOutMax=[]  FilterDiffOutCoefMin=[]  FilterDiffOutCoefMax=[]  ReciprocalOutMin=[]  ReciprocalOutMax=[]  SumDenOutMin=[]  SumDenOutMax=[]  SumNumOutMin=[]  SumNumOutMax=[]  DivideOutMin=[]  DivideOutMax=[]  UdiffTsProdOutMin=[]  UdiffTsProdOutMax=[]  NTsProdOutMin=[]  NTsProdOutMax=[]  UintegralTsProdOutMin=[]  UintegralTsProdOutMax=[]  UngainTsProdOutMin=[]  UngainTsProdOutMax=[]  IntegratorContinuousStateAttributes=''  IntegratorStateMustResolveToSignalObject=off  IntegratorRTWStateStorageClass=Auto  FilterContinuousStateAttributes=''  FilterStateMustResolveToSignalObject=off  FilterRTWStateStorageClass=Auto  ParallelPVariant=InternalParameters  IdealPVariant=Disabled  IVariant=InternalParameters  DVariant=Disabled  IntegratorVariant=Continuous  SatVariant=Disabled  AWVariant=Passthrough  PCopyVariant=Disabled  TRVariant=Disabled  FdbkBlocksVariant=Forward  IdealPFdbkVariant=Disabled  SatFdbkVariant=Disabled  DerivativeFilterVariant=Disabled  NVariant=Disabled  NCopyVariant=Disabled_SignalSpec  FilterICVariant=Disabled  IntegratorICVariant=InternalICs  ExternalResetVariant=Disabled  TRSumVariant=Passthrough  SumFdbkVariant=Disabled  SumVariant=Sum_PI  TsampFilterVariant=InternalTs  TsampNgainVariant=Passthrough  TsampIntegralVariant=Passthrough
  PI Controller for z axis : simulink/Continuous/PID Controller  Controller=PI  Form=Parallel  TimeDomain=Continuous-time  UseExternalTs=off  SampleTime=-1  IntegratorMethod=Forward Euler  FilterMethod=Forward Euler  ControllerParametersSource=internal  P=PIController.z.P  I=PIController.z.I  D=0  UseFilter=on  N=100  TunerSelectOption=Transfer Function Based (PID Tuner App)  InitialConditionSource=internal  InitialConditionForIntegrator=0  InitialConditionForFilter=0  DifferentiatorICPrevScaledInput=0  ExternalReset=none  TrackingMode=off  Kt=1  LimitOutput=off  UpperSaturationLimit=inf  LowerSaturationLimit=-inf  LinearizeAsGain=on  AntiWindupMode=none  Kb=1  POutMin=[]  POutMax=[]  IOutMin=[]  IOutMax=[]  DOutMin=[]  DOutMax=[]  NOutMin=[]  NOutMax=[]  SumOutMin=[]  SumOutMax=[]  SaturationOutMin=[]  SaturationOutMax=[]  PParamMin=[]  PParamMax=[]  IParamMin=[]  IParamMax=[]  DParamMin=[]  DParamMax=[]  NParamMin=[]  NParamMax=[]  KbParamMin=[]  KbParamMax=[]  KtParamMin=[]  KtParamMax=[]  KbOutMin=[]  KbOutMax=[]  KtOutMin=[]  KtOutMax=[]  IntegratorOutMin=[]  IntegratorOutMax=[]  FilterOutMin=[]  FilterOutMax=[]  SumI1OutMin=[]  SumI1OutMax=[]  SumI2OutMin=[]  SumI2OutMax=[]  SumI3OutMin=[]  SumI3OutMax=[]  SumI4OutMin=[]  SumI4OutMax=[]  SumDOutMin=[]  SumDOutMax=[]  DifferentiatorOutMin=[]  DifferentiatorOutMax=[]  FilterDiffOutCoefMin=[]  FilterDiffOutCoefMax=[]  ReciprocalOutMin=[]  ReciprocalOutMax=[]  SumDenOutMin=[]  SumDenOutMax=[]  SumNumOutMin=[]  SumNumOutMax=[]  DivideOutMin=[]  DivideOutMax=[]  UdiffTsProdOutMin=[]  UdiffTsProdOutMax=[]  NTsProdOutMin=[]  NTsProdOutMax=[]  UintegralTsProdOutMin=[]  UintegralTsProdOutMax=[]  UngainTsProdOutMin=[]  UngainTsProdOutMax=[]  IntegratorContinuousStateAttributes=''  IntegratorStateMustResolveToSignalObject=off  IntegratorRTWStateStorageClass=Auto  FilterContinuousStateAttributes=''  FilterStateMustResolveToSignalObject=off  FilterRTWStateStorageClass=Auto  ParallelPVariant=InternalParameters  IdealPVariant=Disabled  IVariant=InternalParameters  DVariant=Disabled  IntegratorVariant=Continuous  SatVariant=Disabled  AWVariant=Passthrough  PCopyVariant=Disabled  TRVariant=Disabled  FdbkBlocksVariant=Forward  IdealPFdbkVariant=Disabled  SatFdbkVariant=Disabled  DerivativeFilterVariant=Disabled  NVariant=Disabled  NCopyVariant=Disabled_SignalSpec  FilterICVariant=Disabled  IntegratorICVariant=InternalICs  ExternalResetVariant=Disabled  TRSumVariant=Passthrough  SumFdbkVariant=Disabled  SumVariant=Sum_PI  TsampFilterVariant=InternalTs  TsampNgainVariant=Passthrough  TsampIntegralVariant=Passthrough
  SB_deg1 : Goto  Commented=on  GotoTag=gear_pos
  Sum : Sum  Inputs=|++
  Sum{1..4} (4 alike) : Sum  Inputs=|+-
  Terminator1 : Terminator
  Terminator2 : Terminator
  "To Workspace alpha_c " : ToWorkspace  VariableName=alpha_c  SaveFormat=Timeseries  SampleTime=-1
  To Workspace f16_control_DYL : ToWorkspace  VariableName=f16_control_DYL  SaveFormat=Timeseries  SampleTime=-1
  To Workspace f16_control_com_pqr : ToWorkspace  VariableName=f16_control_com_pqr  SaveFormat=Timeseries  SampleTime=-1
  To Workspace f16_control_com_μαβ : ToWorkspace  VariableName=f16_control_comm_mu_alpha_beta  SaveFormat=Timeseries  SampleTime=-1
  To Workspace f16_control_err_pqr : ToWorkspace  VariableName=f16_control_Error_pqr  SaveFormat=Timeseries  SampleTime=-1
  To Workspace f16_control_error_μαβ : ToWorkspace  VariableName=f16_control_Error_mu_alpha_beta  SaveFormat=Timeseries  SampleTime=-1
  To Workspace2 : ToWorkspace  VariableName=f16_control_comm_Vt_Chi_Gamma  SaveFormat=Timeseries  SampleTime=-1
  To Workspace3 : ToWorkspace  VariableName=f16_control_Error_V_chi_gamma  SaveFormat=Timeseries  SampleTime=-1
  To Workspace5 : ToWorkspace  VariableName=f16_control_comm_YZ  SaveFormat=Timeseries  SampleTime=-1
  Transfer Fcn1 : TransferFcn  Numerator=[25]  Denominator=[1 10 25]
  Transfer Fcn2 : TransferFcn  Numerator=[25]  Denominator=[1 10 25]
  Transfer Fcn5 : TransferFcn  Numerator=[25]  Denominator=[1 10 25]
  Vehicle : Subsystem
  beta_c : Constant  Value=0
  pqr NDI Controller : Subsystem  Variant=on  VariantControlMode=Label  VariantControl=Choice  LabelModeActiveChoice=TVC ON
  μαβ NDI Controller : Subsystem
  Plant_Data : Outport
  Env_Data : Outport  Port=2
  wires:
  Aerodynamic1/3(aero_control fast G) -> [NDI_aero_control_fast_G]
  PI Controller for beta/1 -> Mux6/3
  PI Controller for y axis/1 -> Mux9/1
  PI Controller for pitch/1 -> Mux1/2
  Iteration Algorithm V chi gamma/3(alpha_command) -> Bus Creator1/2, "To Workspace alpha_c "/1, IC/1, Mux5/2  "alpha_c"
  IC/1 -> Iteration Algorithm V chi gamma/1(alpha_c)  "α_c (rad)"
  μαβ NDI Controller/2(qc) -> Mux4/2
  Mux4/1 -> Sum1/1, To Workspace f16_control_com_pqr/1  "pqr command (rad/s)"
  Demux6/2 -> PI Controller for alpha/1
  Demux4/2 -> Angle Conversion2/1  "chi error"
  μαβ NDI Controller/1(pc) -> Mux4/1
  Demux1/1 -> PI Controller for Vt/1
  Mux10/1 -> Sum3/1, To Workspace5/1  "YZ command"
  Demux3/3 -> PI Controller for yaw/1
  Demux6/1 -> PI Controller for mu/1
  Angle Conversion/1 -> To Workspace f16_control_err_pqr/1
  Iteration Algorithm V chi gamma/2(mu_command) -> Mux5/1  "mu_c"
  6.4.3加裝向量噴嘴以及減速版打開40度模擬著陸速度為200， 上下偏轉向量噴嘴權重值為5.5，75S/3(h (ft)) -> Sum/1
  Demux1/2 -> PI Controller for Chi/1
  μαβ NDI Controller/4(D) -> Mux11/1
  Demux6/3 -> PI Controller for beta/1
  Sum2/1 -> Demux4/1, Demux1/1  "Vt Chi Gamma err"
  Aerodynamic2/3(aero_control fast G) -> Terminator2/1
  μαβ NDI Controller/6(L) -> Mux11/3
  Demux4/3 -> Angle Conversion3/1  "gamma error"
  6.4.3加裝向量噴嘴以及減速版打開40度模擬著陸速度為200， 上下偏轉向量噴嘴權重值為5.5，75S/2(y (ft)) -> Transfer Fcn5/1
  In Bus Element/1 -> μαβ NDI Controller/3(gravity)
  Mux2/1 -> Sum2/1, To Workspace2/1  "Vt Chi Gamma command"
  Sum4/1 -> Angle Conversion1/1, Demux6/1  "μ,α,β err"
  Mux12/1 -> Sum3/2
  Mux5/1 -> Sum4/1, To Workspace f16_control_com_μαβ/1  "mu alpha beta command (rad)"
  Mux6/1 -> μαβ NDI Controller/2(μαβ dot desire)  "mu alpha beta dot desire"
  PI Controller for Chi/1 -> Mux3/2
  6.4.3加裝向量噴嘴以及減速版打開40度模擬著陸速度為200， 上下偏轉向量噴嘴權重值為5.5，75S/1(Vt (ft/s)) -> Mux2/1, Iteration Algorithm Y Z/1(Vc)
  Iteration Algorithm V chi gamma/4(beta_command) -> Mux5/3, Bus Creator1/1  "beta_c"
  Mux3/1 -> Iteration Algorithm V chi gamma/3(Vt,chi,gamma dot desire)  "Vt Chi Gamma dot desire"
  PI Controller for mu/1 -> Mux6/1
  pqr NDI Controller/4(aileron) -> Bus Creator2/2  "aileron"
  beta_c/1 -> Iteration Algorithm V chi gamma/4(beta_cmd)
  μαβ NDI Controller/5(Y) -> Mux11/2
  Demux3/2 -> PI Controller for pitch/1
  6.4.3加裝向量噴嘴以及減速版打開40度模擬著陸速度為200， 上下偏轉向量噴嘴權重值為5.5，75S/5(LandingGear_position) -> Mux14/3, Mux14/2, Mux14/1  "Landing gear normalized position"
  Demux5/2 -> PI Controller for z axis/1
  PI Controller for yaw/1 -> Mux1/3
  Bus Creator/1 -> Vehicle/1(fadec_cmd)
  Mux9/1 -> Iteration Algorithm Y Z/2(Ydot,Zdot des)  "Y Z dot desire"
  Vehicle/1(PlantData) -> pqr NDI Controller/5(AirData), pqr NDI Controller/4(PlantData), Bus Selector1/1, Bus Selector4/1, Iteration Algorithm V chi gamma/6(AirData), Bus Selector/1, Bus Selector3/1, Aerodynamic1/2(PlantData), Aerodynamic1/3(AirData), μαβ NDI Controller/5(AirData), μαβ NDI Controller/4(PlantData), [PlantData], Plant_Data/1
  pqr NDI Controller/2("TVC_y ") -> Bus Creator/3  "TVC_Y"
  Transfer Fcn2/1 -> Mux2/2
  Aerodynamic1/2(aero_control M) -> [NDI_aero_control_M]
  Aerodynamic2/2(aero_control M) -> Terminator1/1
  Demux3/1 -> PI Controller for roll/1
  Angle Conversion1/1 -> To Workspace f16_control_error_μαβ/1
  Mux11/1 -> To Workspace f16_control_DYL/1  "Drag  Side Force Lift"
  Transfer Fcn1/1 -> Mux2/3
  Demux4/1 -> Mux7/1  "Vt error"
  pqr NDI Controller/1(TVC_z) -> Bus Creator/2  "TVC_Z"
  Bus Selector/2 -> Mux12/2  "<altitude>"
  μαβ NDI Controller/3(rc) -> Mux4/3
  [SB_deg] -> Vehicle/3(" SB_deg")
  Angle Conversion2/1 -> Mux7/2
  PI Controller for Gamma/1 -> Mux3/3
  Transfer Fcn5/1 -> Mux10/1  "yc"
  PI Controller for z axis/1 -> Mux9/2
  PI Controller for alpha/1 -> Mux6/2
  Mux7/1 -> To Workspace3/1
  Demux1/3 -> PI Controller for Gamma/1
  Sum3/1 -> Demux5/1  "YZ err"
  Iteration Algorithm Y Z/1(chi_c) -> Transfer Fcn2/1
  6.4.3加裝向量噴嘴以及減速版打開40度模擬著陸速度為200， 上下偏轉向量噴嘴權重值為5.5，75S/4(speed brake (deg)) -> [SB_deg]
  PI Controller for roll/1 -> Mux1/1
  Angle Conversion3/1 -> Mux7/3
  Sum1/1 -> Angle Conversion/1, Demux3/1  "pqr err"
  [NDI_aero_control_M] -> pqr NDI Controller/1(coef M)
  Iteration Algorithm Y Z/2(gamma_c) -> Transfer Fcn1/1
  Aerodynamic1/1(aero_control F) -> [NDI_aero_control_F]
  Gain/1 -> Mux10/2  "zc"
  [NDI_aero_control_fast_G] -> pqr NDI Controller/2(control g)
  Constant/1 -> Sum/2
  [NDI_aero_control_F] -> μαβ NDI Controller/1(aero F)
  pqr NDI Controller/5(rudder) -> Bus Creator2/3  "rudder"
  Sum/1 -> Gain/1
  Mux1/1 -> pqr NDI Controller/3(pqr dot desire)  "pqr dot desire"
  PI Controller for Vt/1 -> Mux3/1
  Demux5/1 -> PI Controller for y axis/1
  Iteration Algorithm V chi gamma/1(thrust_command) -> Bus Creator/1  "thrust"
  [SB_deg] -> Aerodynamic1/1(SB (deg))
  Mux14/1 -> SB_deg1/1
  pqr NDI Controller/3(elevator) -> Bus Creator2/1  "elevator"
  In Bus Element1/1 -> Vehicle/4(EnvData)
  Bus Selector/1 -> Mux12/1  "<epos>"
  [PlantData] -> Aerodynamic2/2(PlantData)
  Bus Selector1/1 -> Mux16/1  "<p>"
  Bus Selector1/2 -> Mux16/2  "<q>"
  Bus Selector1/3 -> Mux16/3  "<r>"
  Mux16/1 -> pqr NDI Controller/6(p q r), Sum1/2
  In Bus Element2/1 -> Iteration Algorithm V chi gamma/5(gravity)
  Bus Creator1/1 -> Aerodynamic2/3(AirData)
  Aerodynamic2/1(aero_control F) -> Iteration Algorithm V chi gamma/2(aero F)
  Bus Selector3/1 -> Mux17/1  "<Vt>"
  Bus Selector3/2 -> Mux17/2  "<chi>"
  Bus Selector3/3 -> Mux17/3  "<gamma>"
  Mux17/1 -> Sum2/2
  [SB_deg] -> Aerodynamic2/1(SB (deg))
  Bus Selector4/1 -> Mux18/1  "<mu>"
  Bus Selector4/2 -> Mux18/2  "<alpha>"
  Bus Selector4/3 -> Mux18/3  "<beta>"
  Mux18/1 -> Sum4/2
  Bus Creator2/1 -> Vehicle/2(fcs_cmd)
  In Bus Element3/1 -> Env_Data/1

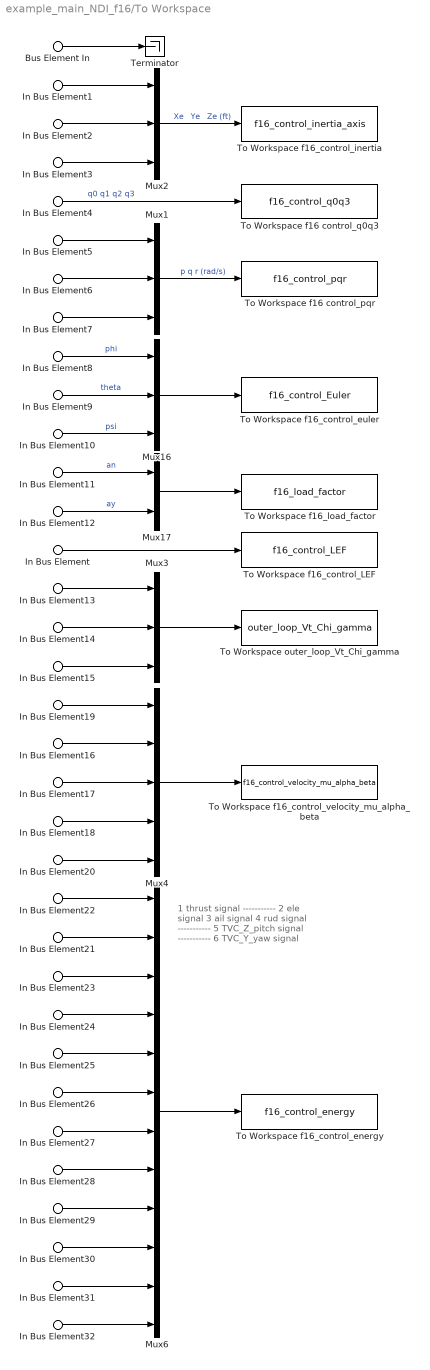
== system example_main_NDI_f16/To Workspace ==
  note: 1 thrust signal
      | -----------
      | 2 ele signal
      | 3 ail signal
      | 4 rud signal
      | -----------
      | 5 TVC_Z_pitch signal
      | -----------
      | 6 TVC_Y_yaw signal
  In Bus Element1 : Inport  PortName=PlantData  Element=npos
  In Bus Element2 : Inport  PortName=PlantData  Element=epos
  In Bus Element3 : Inport  PortName=PlantData  Element=altitude
  In Bus Element4 : Inport  PortName=PlantData  Element=q0q1q2q3
  In Bus Element5 : Inport  PortName=PlantData  Element=p
  In Bus Element6 : Inport  PortName=PlantData  Element=q
  In Bus Element7 : Inport  PortName=PlantData  Element=r
  In Bus Element8 : Inport  PortName=PlantData  Element=phi
  In Bus Element9 : Inport  PortName=PlantData  Element=theta
  In Bus Element10 : Inport  PortName=PlantData  Element=psi
  In Bus Element11 : Inport  PortName=PlantData  Element=an
  In Bus Element12 : Inport  PortName=PlantData  Element=ay
  In Bus Element : Inport  PortName=PlantData  Element=AeroActBus.LEF_deg
  In Bus Element28 : Inport  PortName=PlantData  Element=AeroActBus.Elevator_deg
  In Bus Element29 : Inport  PortName=PlantData  Element=AeroActBus.Aileron_deg
  In Bus Element30 : Inport  PortName=PlantData  Element=AeroActBus.Rudder_deg
  In Bus Element13 : Inport  PortName=PlantData  Element=Vt
  In Bus Element19 : Inport  PortName=PlantData  Element=Vt
  In Bus Element14 : Inport  PortName=PlantData  Element=chi
  In Bus Element15 : Inport  PortName=PlantData  Element=gamma
  In Bus Element20 : Inport  PortName=PlantData  Element=gamma
  In Bus Element16 : Inport  PortName=PlantData  Element=alpha
  In Bus Element17 : Inport  PortName=PlantData  Element=beta
  In Bus Element18 : Inport  PortName=PlantData  Element=mu
  In Bus Element22 : Inport  PortName=PlantData  Element=fadec_cmd.thrust
  In Bus Element25 : Inport  PortName=PlantData  Element=fadec_cmd.TVC_Z
  In Bus Element26 : Inport  PortName=PlantData  Element=fadec_cmd.TVC_Y
  In Bus Element21 : Inport  PortName=PlantData  Element=fcs_cmd.elevator
  In Bus Element23 : Inport  PortName=PlantData  Element=fcs_cmd.aileron
  In Bus Element24 : Inport  PortName=PlantData  Element=fcs_cmd.rudder
  In Bus Element27 : Inport  PortName=PlantData  Element=PropBus.T
  In Bus Element31 : Inport  PortName=PlantData  Element=PropActBus.TVC_Z_pitch_deg
  In Bus Element32 : Inport  PortName=PlantData  Element=PropActBus.TVC_Y_yaw_deg
  Bus Element In : Inport  Port=2  PortName=EnvData
  Mux{1..3,16} (4 alike) : Mux  Inputs=3
  Mux17 : Mux  Inputs=2
  Mux4 : Mux  Inputs=5
  Mux6 : Mux  Inputs=12
  Terminator : Terminator
  To Workspace f16 control_pqr : ToWorkspace  VariableName=f16_control_pqr  SaveFormat=Timeseries  SampleTime=-1
  To Workspace f16 control_q0q3 : ToWorkspace  VariableName=f16_control_q0q3  SaveFormat=Timeseries  SampleTime=-1
  To Workspace f16_control_LEF : ToWorkspace  VariableName=f16_control_LEF  SaveFormat=Timeseries  SampleTime=-1
  To Workspace f16_control_energy : ToWorkspace  VariableName=f16_control_energy  SaveFormat=Timeseries  SampleTime=-1
  To Workspace f16_control_euler : ToWorkspace  VariableName=f16_control_Euler  SaveFormat=Timeseries  SampleTime=-1
  To Workspace f16_control_inertia : ToWorkspace  VariableName=f16_control_inertia_axis  SaveFormat=Timeseries  SampleTime=-1
  To Workspace f16_control_velocity_mu_alpha_beta : ToWorkspace  VariableName=f16_control_velocity_mu_alpha_beta  SaveFormat=Timeseries  SampleTime=-1
  To Workspace f16_load_factor : ToWorkspace  VariableName=f16_load_factor  SaveFormat=Timeseries  SampleTime=-1
  To Workspace outer_loop_Vt_Chi_gamma : ToWorkspace  VariableName=outer_loop_Vt_Chi_gamma  SaveFormat=Timeseries  SampleTime=-1
  wires:
  Mux2/1 -> To Workspace f16_control_inertia/1  "Xe   Ye   Ze (ft)"
  Mux16/1 -> To Workspace f16_control_euler/1
  In Bus Element9/1 -> Mux16/2  "theta"
  In Bus Element10/1 -> Mux16/3  "psi"
  In Bus Element4/1 -> To Workspace f16 control_q0q3/1  "q0 q1 q2 q3"
  In Bus Element11/1 -> Mux17/1  "an"
  In Bus Element8/1 -> Mux16/1  "phi"
  Mux17/1 -> To Workspace f16_load_factor/1
  In Bus Element12/1 -> Mux17/2  "ay"
  Mux1/1 -> To Workspace f16 control_pqr/1  "p q r (rad/s)"
  In Bus Element5/1 -> Mux1/1
  In Bus Element6/1 -> Mux1/2
  In Bus Element7/1 -> Mux1/3
  In Bus Element1/1 -> Mux2/1
  In Bus Element2/1 -> Mux2/2
  In Bus Element3/1 -> Mux2/3
  In Bus Element/1 -> To Workspace f16_control_LEF/1
  In Bus Element13/1 -> Mux3/1
  In Bus Element14/1 -> Mux3/2
  In Bus Element15/1 -> Mux3/3
  Mux3/1 -> To Workspace outer_loop_Vt_Chi_gamma/1
  In Bus Element19/1 -> Mux4/1
  In Bus Element16/1 -> Mux4/2
  In Bus Element17/1 -> Mux4/3
  In Bus Element18/1 -> Mux4/4
  In Bus Element20/1 -> Mux4/5
  Mux4/1 -> To Workspace f16_control_velocity_mu_alpha_beta/1
  In Bus Element22/1 -> Mux6/1
  In Bus Element21/1 -> Mux6/2
  In Bus Element23/1 -> Mux6/3
  In Bus Element24/1 -> Mux6/4
  In Bus Element25/1 -> Mux6/5
  In Bus Element26/1 -> Mux6/6
  In Bus Element27/1 -> Mux6/7
  In Bus Element28/1 -> Mux6/8
  In Bus Element29/1 -> Mux6/9
  In Bus Element30/1 -> Mux6/10
  In Bus Element31/1 -> Mux6/11
  In Bus Element32/1 -> Mux6/12
  Mux6/1 -> To Workspace f16_control_energy/1
  Bus Element In/1 -> Terminator/1
